simulink model "vvc1phase_simpower"  (Simulink 10.2)
settings: Solver=ode3  StartTime=0.0  StopTime=0.5  FixedStep=.00000005  MaxStep=.0000001  RelTol=1e-3  EnableMultiTasking=on
libraries: powerlib x32, simulink x11
(part 1 of 2)
settings Model: Creator=100004357  LastModifiedBy=bjeppese
settings DataIOCC: LimitDataPoints=on
settings OptimizationCC: ExpressionDepthLimit=2147483647
settings DebuggingCC: SolverPrmCheckMsg=warning  MultiTaskDSMMsg=warning  MultiTaskCondExecSysMsg=none  StateNameClashWarn=warning
settings SimscapeCC: SimscapeNormalizeSystem=off

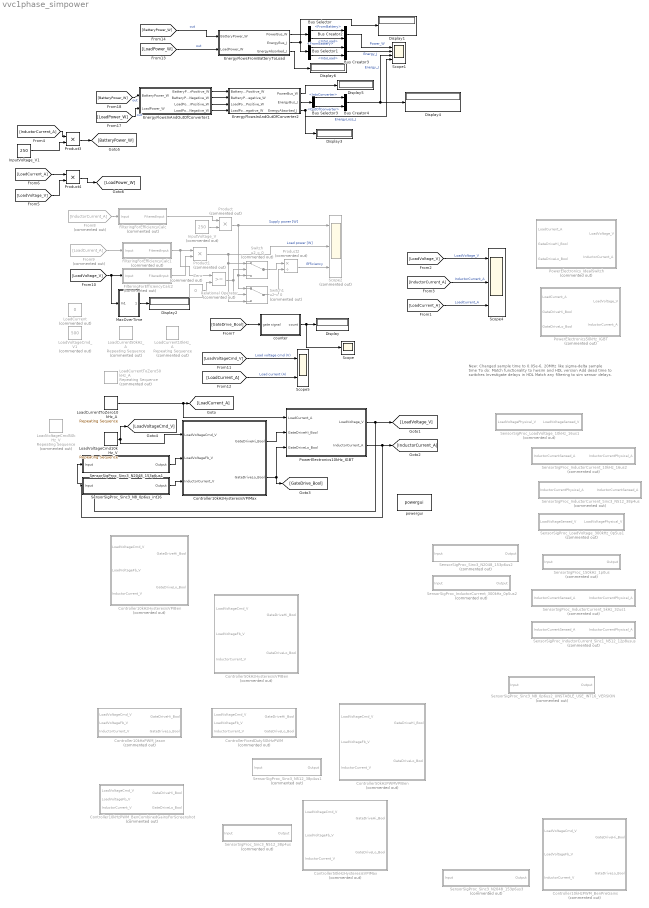
== system vvc1phase_simpower ==
  note: New:
      | Changed sample time to 0.05e-6, 20MHz like sigma-delta sample time
      |
      |
      | To do:
      | Match functionality to hwsim and HDL version
      | Add dead time to switches
      | Investigate delays in HDL
      | Match any filtering to sim sensor delays.
  Bus Creator2 : BusCreator  Inputs=2
  Bus Creator3 : BusCreator  Inputs=2
  Bus Creator4 : BusCreator  Inputs=2
  Bus Selector : BusSelector  OutputSignals=FromBattery,IntoLoad
  Bus Selector1 : BusSelector  OutputSignals=FromBattery,IntoLoad
  Bus Selector3 : BusSelector  OutputSignals=IntoConverter,OutOfConverter
  Controller10kHzHysteresisVPIBen : Subsystem  Commented=on
  Controller10kHzHysteresisVPIMax : Subsystem
  Controller10kHzPWM_BenCombinedGainsForScreenshot : Subsystem  Commented=on
  Controller10kHzPWM_BenPreGains : Subsystem  Commented=on
  "Controller10kHzPWM_Jason " : Subsystem  Commented=on
  Controller50kHzHysteresisVPIBen : Subsystem  Commented=on
  Controller50kHzHysteresisVPIMax : Subsystem  Commented=on
  Controller50kHzPWMVPIBen : Subsystem  Commented=on
  ControllerFixedDuty50kHzPWM : Subsystem  Commented=on
  Display{,1..6} (7 alike) : Display
  EnergyFlowsFromBatteryToLoad : Subsystem
  EnergyFlowsInAndOutOfConverter1 : Subsystem
  EnergyFlowsInAndOutOfConverter2 : Subsystem
  FilteringForEfficiencyCalc : Subsystem  Commented=on
  FilteringForEfficiencyCalc1 : Subsystem  Commented=on
  FilteringForEfficiencyCalc2 : Subsystem  Commented=on
  From8 : From  Commented=on  GotoTag=InductorCurrent_A
  From9 : From  Commented=on  GotoTag=LoadCurrent_A
  InputVoltage_V : Constant  Commented=on  Value=250
  InputVoltage_V1 : Constant  Value=250
  LoadCurrent : Constant  Commented=on  Value=0
  LoadCurrent10kHz_A : simulink/Sources/Repeating Sequence  Commented=on  rep_seq_t=[0 .05 .05001 .100 .10001 .150 .15001 .200 .20001 .250 .25001 .300 .30001 .350 .35001 .400 .40001 .50]  rep_seq_y=[0 0 10 10 -10 -10 20 20 -20 -20 50 50 -50 -50 100 100 -100 -100]
  LoadCurrent50kHz_A : simulink/Sources/Repeating Sequence  Commented=on  rep_seq_t=[0 .01 .01001 .020 .02001 .030 .03001 .040 .04001 .050 .05001 .060 .06001 .070 .07001 .080 .08001 .10]  rep_seq_y=[0 0 10 10 -10 -10 20 20 -20 -20 50 50 -50 -50 100 100 -100 -100]
  LoadCurrentToZero10kHz_A : simulink/Sources/Repeating Sequence  rep_seq_t=[0 .05 .05001 .100 .10001 .150 .15001 .200 .20001 .250 .25001 .300 .30001 .350 .35001 .400 .40001 .450 .45001 .50]  rep_seq_y=[0 0 10 10 -10 -10 20 20 -20 -20 50 50 -50 -50 100 100 -100 -100 0 0]
  LoadCurrentToZero50kHz_A : simulink/Sources/Repeating Sequence  Commented=on  rep_seq_t=[0 .01 .01001 .020 .02001 .030 .03001 .040 .04001 .050 .05001 .060 .06001 .070 .07001 .080 .08001 .090 .09001 .10]  rep_seq_y=[0 0 10 10 -10 -10 20 20 -20 -20 50 50 -50 -50 100 100 -100 -100 0 0]
  LoadVoltageCmd10kHz_V : simulink/Sources/Repeating Sequence  rep_seq_t=[0 0.00501 0.00502 .450 .45001 .50]  rep_seq_y=[250 250 500 500 250 250]
  LoadVoltageCmd50kHz_V : simulink/Sources/Repeating Sequence  Commented=on  rep_seq_t=[0 0.00101 0.00102 .090 .09001 .10]  rep_seq_y=[250 250 500 500 250 250]
  LoadVoltageCmd_V1 : Constant  Commented=on  Value=500
  MaxOverTime : Subsystem
  PowerElectronics10kHz_IGBT : Subsystem
  PowerElectronics50kHz_IGBT : Subsystem  Commented=on
  PowerElectronics_IdealSwitch : Subsystem  Commented=on
  Product : Product  Commented=on
  Product1 : Product  Commented=on
  Product2 : Product  Commented=on  Inputs=*/
  Product3 : Product
  Product4 : Product
  Relational Operator : RelationalOperator  Commented=on  OutDataTypeStr=boolean  RndMeth=Nearest
  Scope : Scope
  Scope1 : Scope  NumInputPorts=4
  Scope2 : Scope  Commented=on  NumInputPorts=3
  Scope4 : Scope  NumInputPorts=3
  Scope5 : Scope  NumInputPorts=2
  SensorSigProc_150kHz_1p0us : Subsystem  Commented=on
  SensorSigProc_InductorCurrent_10kHz_16us2 : Subsystem  Commented=on
  SensorSigProc_InductorCurrent_300kHz_0p5us2 : Subsystem  Commented=on
  SensorSigProc_InductorCurrent_5kHz_32us1 : Subsystem  Commented=on
  SensorSigProc_InductorCurrent_Sinc1_N512_12p8usus : Subsystem  Commented=on
  SensorSigProc_InductorCurrent_Sinc3_N512_38p4us : Subsystem  Commented=on
  SensorSigProc_LoadVoltage_10kHz_16us1 : Subsystem  Commented=on
  SensorSigProc_LoadVoltage_300kHz_0p5us1 : Subsystem  Commented=on
  SensorSigProc_Sinc3_N2048_153p6us1 : Subsystem
  SensorSigProc_Sinc3_N2048_153p6us2 : Subsystem  Commented=on
  SensorSigProc_Sinc3_N2048_153p6us3 : Subsystem  Commented=on
  SensorSigProc_Sinc3_N512_38p4us : Subsystem  Commented=on
  SensorSigProc_Sinc3_N512_38p4us1 : Subsystem  Commented=on
  SensorSigProc_Sinc3_N8_0p6us2_UNSTABLE_USE_INT16_VERSION : Subsystem  Commented=on
  SensorSigProc_Sinc3_N8_0p6us_int16 : Subsystem
  Switch : Switch  Commented=on  Criteria=u2 > Threshold
  Switch1 : Switch  Commented=on  Criteria=u2 > Threshold
  Zero : Constant  Commented=on  Value=0
  "counter " : Subsystem
  powergui : powerlib/powergui  Priority=1  SimulationMode=Discrete  SampleTime=5e-8  frequency=60  Iterations=50  frequencyindice=0  Pbase=100e6  ErrMax=1e-4  UnitsV=kV  UnitsW=MW  buscounter=0  FunctionMessages=off  echomessages=off  EnableUseOfTLC=off  CurrentSourceSwitches=off  DisableSnubberDevices=off  DisableRonSwitches=off  DisableVfSwitches=off  DisplayEquations=off  AutomaticDiscreteSolvers=off  SolverType=Tustin  Interpol=off  ExternalGateDelay=off  methode=off  Ts=0  x0status=blocks  SPID=off  SwTol=0  HookPort=off  NonlinearTolerance=1e-4  nMaxIteration=100  ContinueOnMaxIteration=off  RestoreLinks=warning  ResistiveCurrentMeasurement=off  Frange=[0:2:500]  Ylog=off  Xlog=on  ShowGrid=off  save=off  variable=ZData  structure=0  ZoomFFT=off  StartTime=0.0  cycles=1  DisplayStyle=1  fundamental=60  FreqAxis=off  MaxFrequency=1000  frequencyindicesteady=1  RmsSteady=1  display=off
  wires:
  From8/1 -> FilteringForEfficiencyCalc/1(Input)
  InputVoltage_V/1 -> Product/2
  Product/1 -> Switch1/1, Switch/3, Scope2/1  "Supply power [W]"
  From9/1 -> FilteringForEfficiencyCalc1/1(Input)
  [LoadVoltage_V] -> MaxOverTime/1(In1), FilteringForEfficiencyCalc2/1(Input)
  Product1/1 -> Switch1/3, Switch/1, Scope2/2  "Load power [W]"
  Product2/1 -> Scope2/3  "Efficiency"
  LoadVoltageCmd10kHz_V/1 -> Controller10kHzHysteresisVPIMax/1(LoadVoltageCmd_V), [LoadVoltageCmd_V]
  PowerElectronics10kHz_IGBT/1(LoadVoltage_V) -> SensorSigProc_Sinc3_N2048_153p6us1/1(Input), [LoadVoltage_V]
  PowerElectronics10kHz_IGBT/2(InductorCurrent_A) -> SensorSigProc_Sinc3_N8_0p6us_int16/1(Input), [InductorCurrent_A]
  [LoadCurrent_A] -> Scope4/3  "LoadCurrent_A"
  [LoadVoltage_V] -> Scope4/1  "LoadVoltage_V"
  [InductorCurrent_A] -> Scope4/2  "InductorCurrent_A"
  FilteringForEfficiencyCalc/1(FiteredInput) -> Product/1
  FilteringForEfficiencyCalc1/1(FiteredInput) -> Relational Operator/1, Product1/1
  FilteringForEfficiencyCalc2/1(FiteredInput) -> Product1/2
  Controller10kHzHysteresisVPIMax/2(GateDriveLo_Bool) -> [GateDrive_Bool], PowerElectronics10kHz_IGBT/3(GateDriveLo_Bool)
  Zero/1 -> Relational Operator/2
  Relational Operator/1 -> Switch/2, Switch1/2
  Switch/1 -> Product2/1
  Switch1/1 -> Product2/2
  LoadCurrentToZero10kHz_A/1 -> PowerElectronics10kHz_IGBT/1(LoadCurrent_A), [LoadCurrent_A]
  "counter "/1(count) -> Scope/1, Display/1
  [GateDrive_Bool] -> "counter "/1(gate signal)
  Controller10kHzHysteresisVPIMax/1(GateDriveHi_Bool) -> PowerElectronics10kHz_IGBT/2(GateDriveHi_Bool)
  SensorSigProc_Sinc3_N2048_153p6us1/1(Output) -> Controller10kHzHysteresisVPIMax/2(LoadVoltageFb_V)
  SensorSigProc_Sinc3_N8_0p6us_int16/1(Output) -> Controller10kHzHysteresisVPIMax/3(InductorCurrent_V)
  [LoadVoltageCmd_V] -> Scope5/1  "Load voltage cmd (V)"
  [LoadCurrent_A] -> Scope5/2  "Load current (A)"
  [LoadCurrent_A] -> Product4/1
  [LoadVoltage_V] -> Product4/2
  Product4/1 -> [LoadPower_W]
  InputVoltage_V1/1 -> Product3/2
  [InductorCurrent_A] -> Product3/1
  Product3/1 -> [BatteryPower_W]
  EnergyFlowsFromBatteryToLoad/2(EnergyBus_J) -> Bus Selector1/1, Display1/1
  [BatteryPower_W] -> EnergyFlowsFromBatteryToLoad/1(BatteryPower_W)  "out"
  [LoadPower_W] -> EnergyFlowsFromBatteryToLoad/2(LoadPower_W)  "out"
  [BatteryPower_W] -> EnergyFlowsInAndOutOfConverter1/1(BatteryPower_W)  "out"
  [LoadPower_W] -> EnergyFlowsInAndOutOfConverter1/2(LoadPower_W)  "out"
  EnergyFlowsInAndOutOfConverter1/4(LoadPowerNegative_W) -> EnergyFlowsInAndOutOfConverter2/4(LoadPowerNegative_W)
  EnergyFlowsInAndOutOfConverter1/1(BatteryPowerPositive_W) -> EnergyFlowsInAndOutOfConverter2/1(BatteryPowerPositive_W)
  EnergyFlowsInAndOutOfConverter1/2(BatteryPowerNegative_W) -> EnergyFlowsInAndOutOfConverter2/2(BatteryPowerNegative_W)
  EnergyFlowsInAndOutOfConverter1/3(LoadPowerPositive_W) -> EnergyFlowsInAndOutOfConverter2/3(LoadPowerPositive_W)
  EnergyFlowsFromBatteryToLoad/1(PowerBus_W) -> Bus Selector/1
  Bus Selector/2 -> Bus Creator2/2  "<IntoLoad>"
  Bus Selector/1 -> Bus Creator2/1  "<FromBattery>"
  Bus Creator2/1 -> Scope1/1  "Power_W"
  Bus Selector1/1 -> Bus Creator3/1  "<FromBattery>"
  Bus Selector1/2 -> Bus Creator3/2  "<IntoLoad>"
  Bus Creator3/1 -> Scope1/2  "Energy_J"
  EnergyFlowsInAndOutOfConverter2/2(EnergyBus_J) -> Bus Selector3/1
  Bus Selector3/2 -> Bus Creator4/2  "<OutOfConverter>"
  Bus Creator4/1 -> Scope1/3, Display4/1  "Energy_J"
  Bus Selector3/1 -> Bus Creator4/1  "<IntoConverter>"
  EnergyFlowsInAndOutOfConverter2/3(EnergyAbsorbed_J) -> Scope1/4, Display3/1  "EnergyLoss_J"
  EnergyFlowsInAndOutOfConverter2/1(PowerBus_W) -> Display5/1
  EnergyFlowsFromBatteryToLoad/3(EnergyAbsorbed_J) -> Display6/1
  MaxOverTime/1(Out1) -> Display2/1

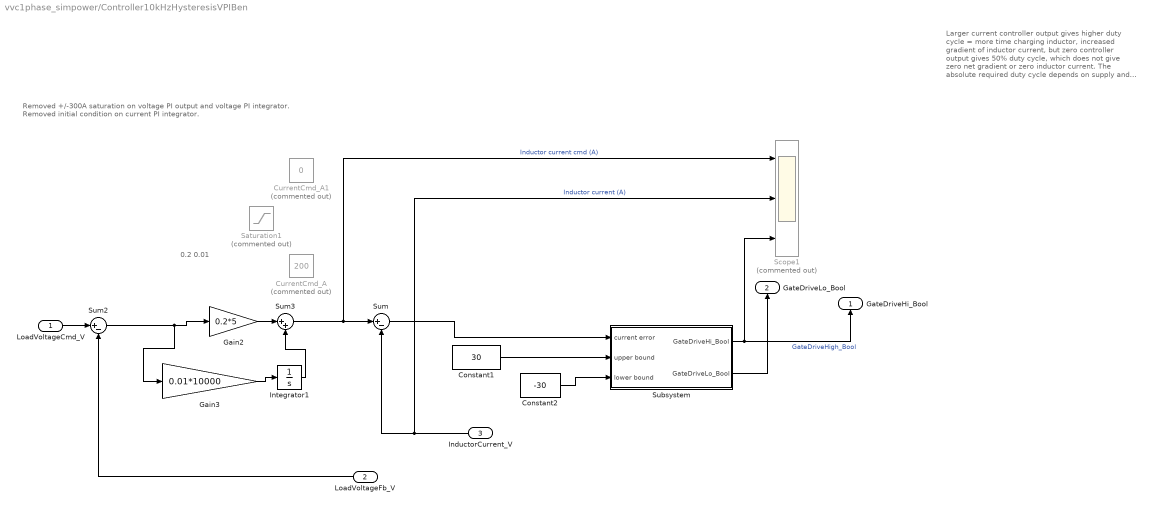
== system vvc1phase_simpower/Controller10kHzHysteresisVPIBen ==
  note: Removed +/-300A saturation on voltage PI output and voltage PI integrator.
      | Removed initial condition on current PI integrator.
  note: Larger current controller output gives higher duty
      | cycle = more time charging inductor,
      | increased gradient of inductor current,
      | but zero controller output gives 50% duty cycle,
      | which does not give zero net gradient
      | or zero inductor current.
      |
      | The absolute required duty cycle depends on
      | supply and load voltages (known)
      | and load current  (unknown)
      | as well as inductor current error.
      |
      | On switch on, with 250V at supply and load,
      | a minimum duty cycle (-0.99) is required to
      | achieve an initial zero inductor current.
      |
      | If zero (50%) were applied initially,
      | inductor current will quickly rise because there
      | is no net voltage reducing it when the inductor
      | is connector to the load. The integrator initial
      | value is used to achieve this.
      |
      | Once the 500V load voltage demand is applied,
      | the voltage controller will give a positive
      | inductor current command.
      | the current P and I gains will raise the duty cycle
      | and the integrator will rise towards zero.
      |
      | Current controller tends to oscillate because
      | controller output only affects gradient of
      | inductor current. Would probably be better
      | with a derivative term
  note: 0.2
      | 0.01
  LoadVoltageCmd_V : Inport
  LoadVoltageFb_V : Inport  Port=2
  InductorCurrent_V : Inport  Port=3
  Constant1 : Constant  Value=30
  Constant2 : Constant  Value=-30
  CurrentCmd_A : Constant  Commented=on  Value=200
  CurrentCmd_A1 : Constant  Commented=on  Value=0
  Gain2 : Gain  Gain=0.2*5
  Gain3 : Gain  Gain=0.01*10000
  Integrator1 : Integrator  UpperSaturationLimit=300  LowerSaturationLimit=-300
  Saturation1 : Saturate  Commented=on  UpperLimit=300  LowerLimit=-300
  Scope1 : Scope  Commented=on  NumInputPorts=3
  Subsystem : Subsystem
  Sum : Sum  Inputs=|+-
  Sum2 : Sum  Inputs=|+-
  Sum3 : Sum  Inputs=|++
  GateDriveHi_Bool : Outport
  GateDriveLo_Bool : Outport  Port=2
  wires:
  Sum3/1 -> Scope1/1, Sum/1  "Inductor current cmd (A)"
  Sum2/1 -> Gain3/1, Gain2/1
  Sum/1 -> Subsystem/1(current error)
  Gain3/1 -> Integrator1/1
  LoadVoltageCmd_V/1 -> Sum2/1
  Integrator1/1 -> Sum3/2
  LoadVoltageFb_V/1 -> Sum2/2
  InductorCurrent_V/1 -> Scope1/2, Sum/2  "Inductor current (A)"
  Gain2/1 -> Sum3/1
  Constant2/1 -> Subsystem/3(lower bound)
  Constant1/1 -> Subsystem/2(upper bound)
  Subsystem/1(GateDriveHi_Bool) -> Scope1/3, GateDriveHi_Bool/1  "GateDriveHigh_Bool"
  Subsystem/2(GateDriveLo_Bool) -> GateDriveLo_Bool/1

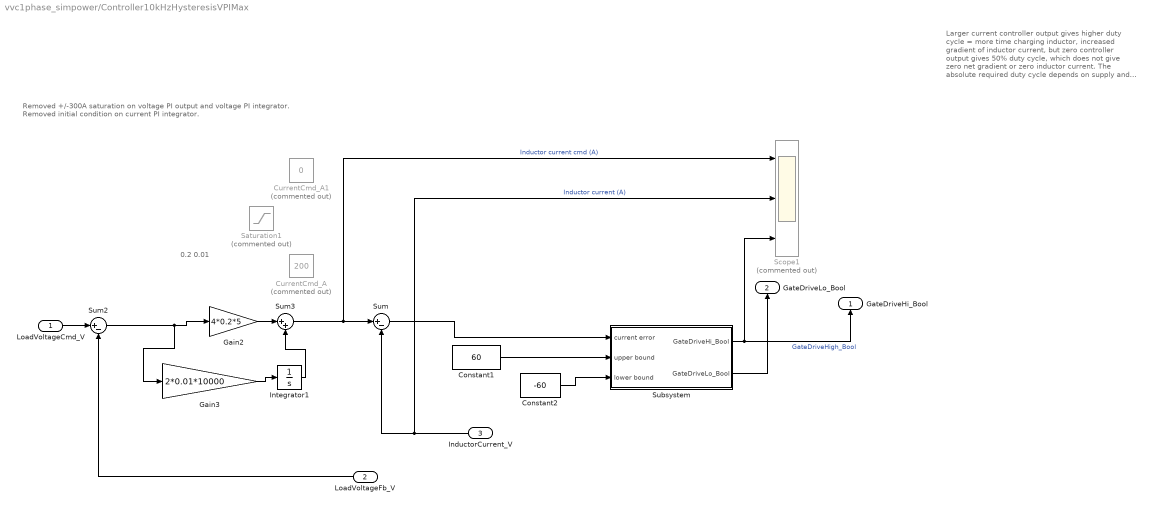
== system vvc1phase_simpower/Controller10kHzHysteresisVPIMax ==
  note: 0.2
      | 0.01
  note: Larger current controller output gives higher duty
      | cycle = more time charging inductor,
      | increased gradient of inductor current,
      | but zero controller output gives 50% duty cycle,
      | which does not give zero net gradient
      | or zero inductor current.
      |
      | The absolute required duty cycle depends on
      | supply and load voltages (known)
      | and load current  (unknown)
      | as well as inductor current error.
      |
      | On switch on, with 250V at supply and load,
      | a minimum duty cycle (-0.99) is required to
      | achieve an initial zero inductor current.
      |
      | If zero (50%) were applied initially,
      | inductor current will quickly rise because there
      | is no net voltage reducing it when the inductor
      | is connector to the load. The integrator initial
      | value is used to achieve this.
      |
      | Once the 500V load voltage demand is applied,
      | the voltage controller will give a positive
      | inductor current command.
      | the current P and I gains will raise the duty cycle
      | and the integrator will rise towards zero.
      |
      | Current controller tends to oscillate because
      | controller output only affects gradient of
      | inductor current. Would probably be better
      | with a derivative term
  note: Removed +/-300A saturation on voltage PI output and voltage PI integrator.
      | Removed initial condition on current PI integrator.
  LoadVoltageCmd_V : Inport
  LoadVoltageFb_V : Inport  Port=2
  InductorCurrent_V : Inport  Port=3
  Constant1 : Constant  Value=60
  Constant2 : Constant  Value=-60
  CurrentCmd_A : Constant  Commented=on  Value=200
  CurrentCmd_A1 : Constant  Commented=on  Value=0
  Gain2 : Gain  Gain=4*0.2*5
  Gain3 : Gain  Gain=2*0.01*10000
  Integrator1 : Integrator  UpperSaturationLimit=300  LowerSaturationLimit=-300
  Saturation1 : Saturate  Commented=on  UpperLimit=300  LowerLimit=-300
  Scope1 : Scope  Commented=on  NumInputPorts=3
  Subsystem : Subsystem
  Sum : Sum  Inputs=|+-
  Sum2 : Sum  Inputs=|+-
  Sum3 : Sum  Inputs=|++
  GateDriveHi_Bool : Outport
  GateDriveLo_Bool : Outport  Port=2
  wires:
  Subsystem/2(GateDriveLo_Bool) -> GateDriveLo_Bool/1
  Subsystem/1(GateDriveHi_Bool) -> GateDriveHi_Bool/1, Scope1/3  "GateDriveHigh_Bool"
  Constant1/1 -> Subsystem/2(upper bound)
  Constant2/1 -> Subsystem/3(lower bound)
  Gain2/1 -> Sum3/1
  InductorCurrent_V/1 -> Sum/2, Scope1/2  "Inductor current (A)"
  LoadVoltageFb_V/1 -> Sum2/2
  Integrator1/1 -> Sum3/2
  LoadVoltageCmd_V/1 -> Sum2/1
  Gain3/1 -> Integrator1/1
  Sum/1 -> Subsystem/1(current error)
  Sum2/1 -> Gain2/1, Gain3/1
  Sum3/1 -> Sum/1, Scope1/1  "Inductor current cmd (A)"

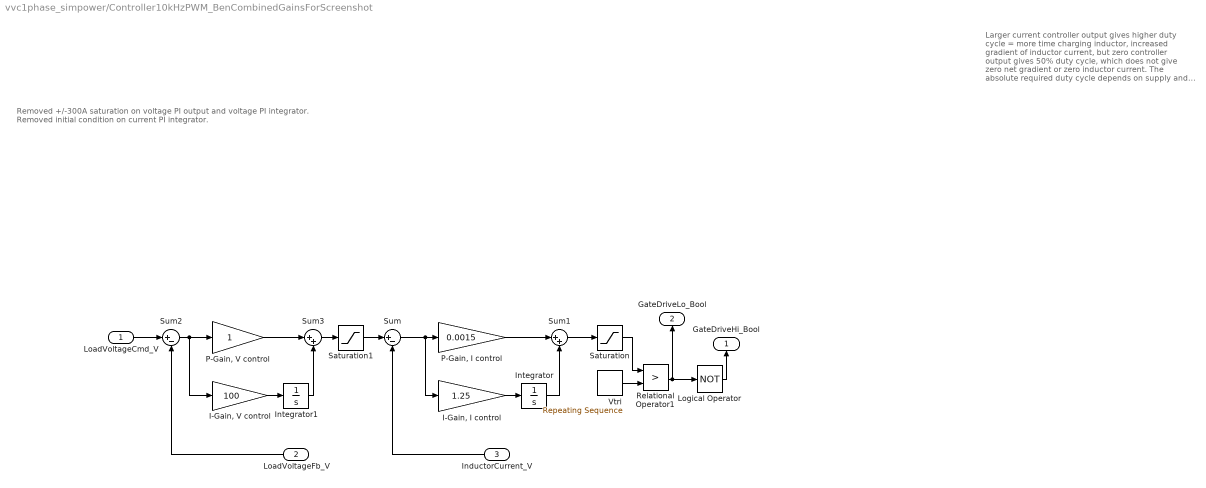
== system vvc1phase_simpower/Controller10kHzPWM_BenCombinedGainsForScreenshot ==
  note: Removed +/-300A saturation on voltage PI output and voltage PI integrator.
      | Removed initial condition on current PI integrator.
  note: Larger current controller output gives higher duty
      | cycle = more time charging inductor,
      | increased gradient of inductor current,
      | but zero controller output gives 50% duty cycle,
      | which does not give zero net gradient
      | or zero inductor current.
      |
      | The absolute required duty cycle depends on
      | supply and load voltages (known)
      | and load current  (unknown)
      | as well as inductor current error.
      |
      | On switch on, with 250V at supply and load,
      | a minimum duty cycle (-0.99) is required to
      | achieve an initial zero inductor current.
      |
      | If zero (50%) were applied initially,
      | inductor current will quickly rise because there
      | is no net voltage reducing it when the inductor
      | is connector to the load. The integrator initial
      | value is used to achieve this.
      |
      | Once the 500V load voltage demand is applied,
      | the voltage controller will give a positive
      | inductor current command.
      | the current P and I gains will raise the duty cycle
      | and the integrator will rise towards zero.
      |
      | Current controller tends to oscillate because
      | controller output only affects gradient of
      | inductor current. Would probably be better
      | with a derivative term
  LoadVoltageCmd_V : Inport
  LoadVoltageFb_V : Inport  Port=2
  InductorCurrent_V : Inport  Port=3
  "I-Gain, I control" : Gain  Gain=1.25
  "I-Gain, V control" : Gain  Gain=100
  Integrator : Integrator  InitialCondition=-0.99  LimitOutput=on  UpperSaturationLimit=.99  LowerSaturationLimit=-.99
  Integrator1 : Integrator  LimitOutput=on  UpperSaturationLimit=300  LowerSaturationLimit=-300
  Logical Operator : Logic  Operator=NOT  AllPortsSameDT=off  OutDataTypeStr=boolean
  "P-Gain, I control" : Gain  Gain=0.0015
  "P-Gain, V control" : Gain
  Relational Operator1 : RelationalOperator  Operator=>  OutDataTypeStr=boolean  RndMeth=Nearest
  Saturation : Saturate  UpperLimit=.99  LowerLimit=-.99
  Saturation1 : Saturate  UpperLimit=300  LowerLimit=-300
  Sum : Sum  Inputs=|+-
  Sum1 : Sum  Inputs=|++
  Sum2 : Sum  Inputs=|+-
  Sum3 : Sum  Inputs=|++
  Vtri : simulink/Sources/Repeating Sequence  rep_seq_t=[0 1/20000 1/10000 ]  rep_seq_y=[-1 1 -1]
  GateDriveHi_Bool : Outport
  GateDriveLo_Bool : Outport  Port=2
  wires:
  Sum3/1 -> Saturation1/1
  Sum2/1 -> "P-Gain, V control"/1, "I-Gain, V control"/1
  Sum/1 -> "I-Gain, I control"/1, "P-Gain, I control"/1
  "I-Gain, V control"/1 -> Integrator1/1
  Logical Operator/1 -> GateDriveHi_Bool/1
  LoadVoltageCmd_V/1 -> Sum2/1
  Integrator1/1 -> Sum3/2
  Integrator/1 -> Sum1/2
  "I-Gain, I control"/1 -> Integrator/1
  Relational Operator1/1 -> Logical Operator/1, GateDriveLo_Bool/1
  "P-Gain, I control"/1 -> Sum1/1
  Saturation/1 -> Relational Operator1/1
  Sum1/1 -> Saturation/1
  LoadVoltageFb_V/1 -> Sum2/2
  InductorCurrent_V/1 -> Sum/2
  Vtri/1 -> Relational Operator1/2
  "P-Gain, V control"/1 -> Sum3/1
  Saturation1/1 -> Sum/1

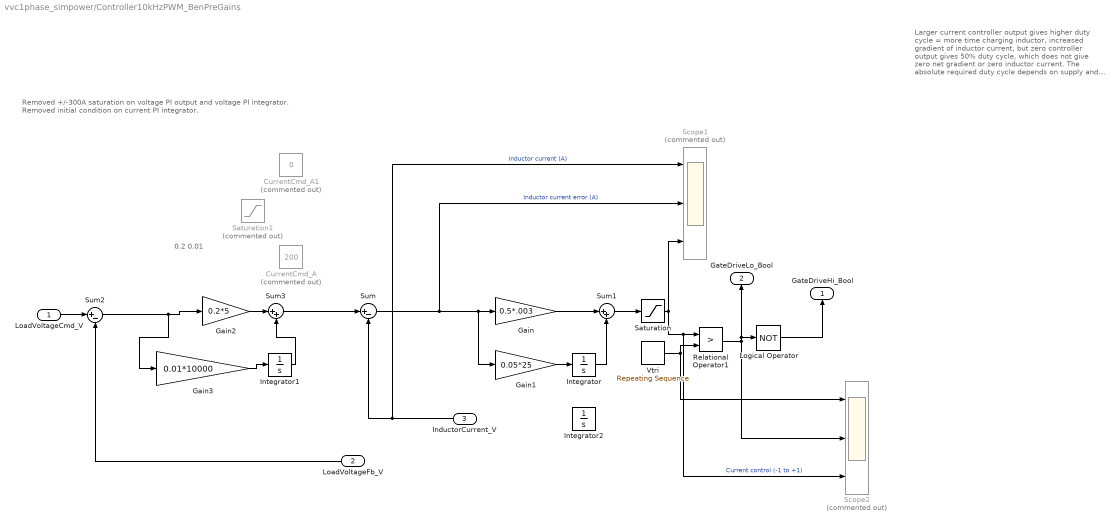
== system vvc1phase_simpower/Controller10kHzPWM_BenPreGains ==
  note: 0.2
      | 0.01
  note: Larger current controller output gives higher duty
      | cycle = more time charging inductor,
      | increased gradient of inductor current,
      | but zero controller output gives 50% duty cycle,
      | which does not give zero net gradient
      | or zero inductor current.
      |
      | The absolute required duty cycle depends on
      | supply and load voltages (known)
      | and load current  (unknown)
      | as well as inductor current error.
      |
      | On switch on, with 250V at supply and load,
      | a minimum duty cycle (-0.99) is required to
      | achieve an initial zero inductor current.
      |
      | If zero (50%) were applied initially,
      | inductor current will quickly rise because there
      | is no net voltage reducing it when the inductor
      | is connector to the load. The integrator initial
      | value is used to achieve this.
      |
      | Once the 500V load voltage demand is applied,
      | the voltage controller will give a positive
      | inductor current command.
      | the current P and I gains will raise the duty cycle
      | and the integrator will rise towards zero.
      |
      | Current controller tends to oscillate because
      | controller output only affects gradient of
      | inductor current. Would probably be better
      | with a derivative term
  note: Removed +/-300A saturation on voltage PI output and voltage PI integrator.
      | Removed initial condition on current PI integrator.
  LoadVoltageCmd_V : Inport
  LoadVoltageFb_V : Inport  Port=2
  InductorCurrent_V : Inport  Port=3
  CurrentCmd_A : Constant  Commented=on  Value=200
  CurrentCmd_A1 : Constant  Commented=on  Value=0
  Gain : Gain  Gain=0.5*.003
  Gain1 : Gain  Gain=0.05*25
  Gain2 : Gain  Gain=0.2*5
  Gain3 : Gain  Gain=0.01*10000
  Integrator : Integrator  InitialCondition=-0.99  LimitOutput=on  UpperSaturationLimit=.99  LowerSaturationLimit=-.99
  Integrator1 : Integrator  UpperSaturationLimit=300  LowerSaturationLimit=-300
  Integrator2 : Integrator  InitialCondition=-.99  LimitOutput=on  UpperSaturationLimit=.99  LowerSaturationLimit=-.99
  Logical Operator : Logic  Operator=NOT  AllPortsSameDT=off  OutDataTypeStr=boolean
  Relational Operator1 : RelationalOperator  Operator=>  OutDataTypeStr=boolean  RndMeth=Nearest
  Saturation : Saturate  UpperLimit=.99  LowerLimit=-.99
  Saturation1 : Saturate  Commented=on  UpperLimit=300  LowerLimit=-300
  Scope1 : Scope  Commented=on  NumInputPorts=3
  Scope2 : Scope  Commented=on  NumInputPorts=3
  Sum : Sum  Inputs=|+-
  Sum1 : Sum  Inputs=|++
  Sum2 : Sum  Inputs=|+-
  Sum3 : Sum  Inputs=|++
  Vtri : simulink/Sources/Repeating Sequence  rep_seq_t=[0 1/20000 1/10000 ]  rep_seq_y=[-1 1 -1]
  GateDriveHi_Bool : Outport
  GateDriveLo_Bool : Outport  Port=2
  wires:
  Gain2/1 -> Sum3/1
  Vtri/1 -> Relational Operator1/2, Scope2/1
  InductorCurrent_V/1 -> Scope1/1, Sum/2  "Inductor current (A)"
  LoadVoltageFb_V/1 -> Sum2/2
  Sum1/1 -> Saturation/1
  Saturation/1 -> Scope1/3, Scope2/3, Relational Operator1/1  "Current control (-1 to +1)"
  Gain/1 -> Sum1/1
  Relational Operator1/1 -> GateDriveLo_Bool/1, Logical Operator/1, Scope2/2
  Gain1/1 -> Integrator/1
  Integrator/1 -> Sum1/2
  Integrator1/1 -> Sum3/2
  LoadVoltageCmd_V/1 -> Sum2/1
  Logical Operator/1 -> GateDriveHi_Bool/1
  Gain3/1 -> Integrator1/1
  Sum/1 -> Scope1/2, Gain1/1, Gain/1  "Inductor current error (A)"
  Sum2/1 -> Gain2/1, Gain3/1
  Sum3/1 -> Sum/1

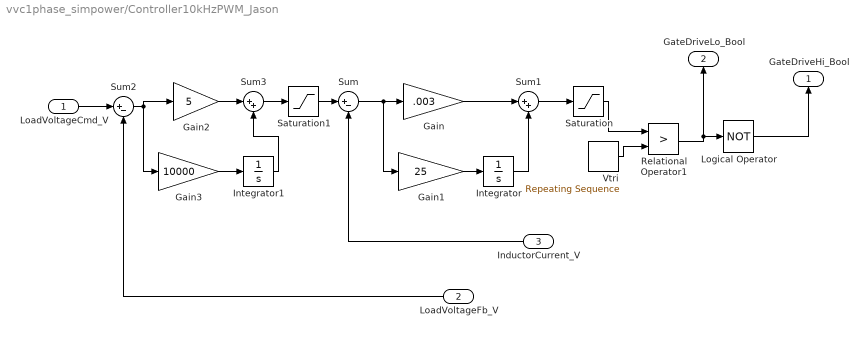
== system vvc1phase_simpower/Controller10kHzPWM_Jason  ==
  LoadVoltageCmd_V : Inport
  LoadVoltageFb_V : Inport  Port=2
  InductorCurrent_V : Inport  Port=3
  Gain : Gain  Gain=.003
  Gain1 : Gain  Gain=25
  Gain2 : Gain  Gain=5
  Gain3 : Gain  Gain=10000
  Integrator : Integrator  InitialCondition=-.99  LimitOutput=on  UpperSaturationLimit=.99  LowerSaturationLimit=-.99
  Integrator1 : Integrator  LimitOutput=on  UpperSaturationLimit=300  LowerSaturationLimit=-300
  Logical Operator : Logic  Operator=NOT  AllPortsSameDT=off  OutDataTypeStr=boolean
  Relational Operator1 : RelationalOperator  Operator=>  OutDataTypeStr=boolean  RndMeth=Nearest
  Saturation : Saturate  UpperLimit=.99  LowerLimit=-.99
  Saturation1 : Saturate  UpperLimit=300  LowerLimit=-300
  Sum : Sum  Inputs=|+-
  Sum1 : Sum  Inputs=|++
  Sum2 : Sum  Inputs=|+-
  Sum3 : Sum  Inputs=|++
  Vtri : simulink/Sources/Repeating Sequence  rep_seq_t=[0 1/20000 1/10000 ]  rep_seq_y=[-1 1 -1]
  GateDriveHi_Bool : Outport
  GateDriveLo_Bool : Outport  Port=2
  wires:
  Gain3/1 -> Integrator1/1
  Logical Operator/1 -> GateDriveHi_Bool/1
  LoadVoltageCmd_V/1 -> Sum2/1
  Integrator1/1 -> Sum3/2
  Integrator/1 -> Sum1/2
  Gain1/1 -> Integrator/1
  Sum2/1 -> Gain2/1, Gain3/1
  Relational Operator1/1 -> GateDriveLo_Bool/1, Logical Operator/1
  Gain/1 -> Sum1/1
  Saturation/1 -> Relational Operator1/1
  Sum1/1 -> Saturation/1
  Saturation1/1 -> Sum/1
  LoadVoltageFb_V/1 -> Sum2/2
  InductorCurrent_V/1 -> Sum/2
  Vtri/1 -> Relational Operator1/2
  Sum/1 -> Gain/1, Gain1/1
  Gain2/1 -> Sum3/1
  Sum3/1 -> Saturation1/1

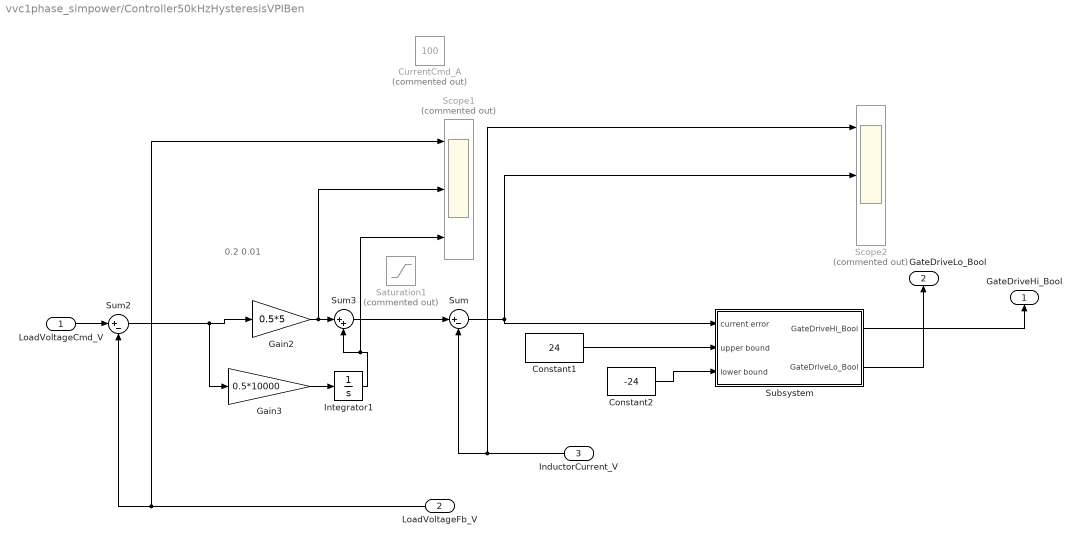
== system vvc1phase_simpower/Controller50kHzHysteresisVPIBen ==
  note: 0.2
      | 0.01
  LoadVoltageCmd_V : Inport
  LoadVoltageFb_V : Inport  Port=2
  InductorCurrent_V : Inport  Port=3
  Constant1 : Constant  Value=24
  Constant2 : Constant  Value=-24
  CurrentCmd_A : Constant  Commented=on  Value=100
  Gain2 : Gain  Gain=0.5*5
  Gain3 : Gain  Gain=0.5*10000
  Integrator1 : Integrator  UpperSaturationLimit=300  LowerSaturationLimit=-300
  Saturation1 : Saturate  Commented=on  UpperLimit=300  LowerLimit=-300
  Scope1 : Scope  Commented=on  NumInputPorts=3
  Scope2 : Scope  Commented=on  NumInputPorts=3
  Subsystem : Subsystem
  Sum : Sum  Inputs=|+-
  Sum2 : Sum  Inputs=|+-
  Sum3 : Sum  Inputs=|++
  GateDriveHi_Bool : Outport
  GateDriveLo_Bool : Outport  Port=2
  wires:
  Subsystem/2(GateDriveLo_Bool) -> GateDriveLo_Bool/1
  Constant1/1 -> Subsystem/2(upper bound)
  Constant2/1 -> Subsystem/3(lower bound)
  Gain2/1 -> Scope1/2, Sum3/1
  InductorCurrent_V/1 -> Scope2/1, Sum/2
  LoadVoltageFb_V/1 -> Scope1/1, Sum2/2
  Integrator1/1 -> Scope1/3, Sum3/2
  LoadVoltageCmd_V/1 -> Sum2/1
  Subsystem/1(GateDriveHi_Bool) -> GateDriveHi_Bool/1
  Gain3/1 -> Integrator1/1
  Sum/1 -> Scope2/2, Subsystem/1(current error)
  Sum2/1 -> Gain2/1, Gain3/1
  Sum3/1 -> Sum/1

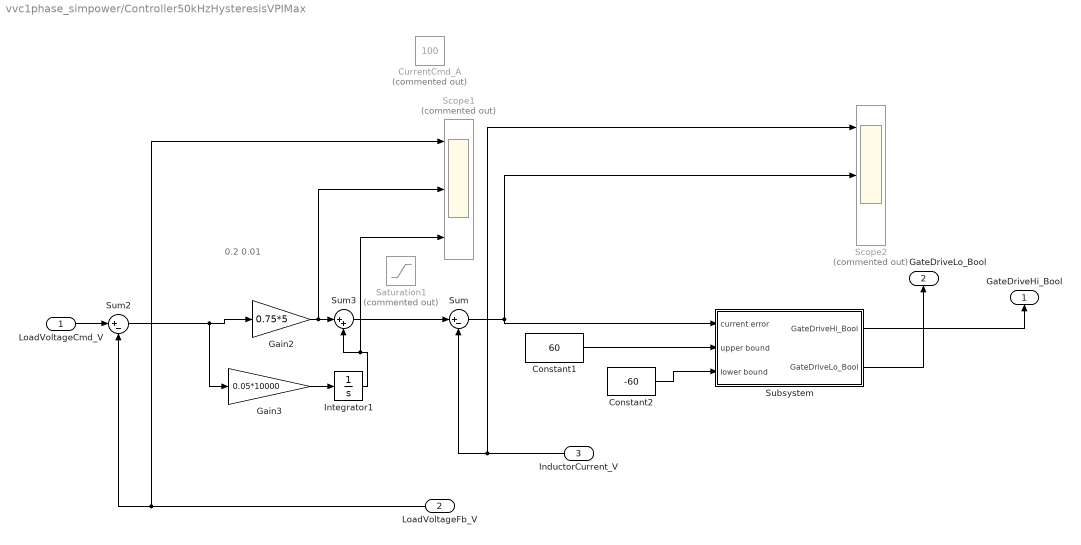
== system vvc1phase_simpower/Controller50kHzHysteresisVPIMax ==
  note: 0.2
      | 0.01
  LoadVoltageCmd_V : Inport
  LoadVoltageFb_V : Inport  Port=2
  InductorCurrent_V : Inport  Port=3
  Constant1 : Constant  Value=60
  Constant2 : Constant  Value=-60
  CurrentCmd_A : Constant  Commented=on  Value=100
  Gain2 : Gain  Gain=0.75*5
  Gain3 : Gain  Gain=0.05*10000
  Integrator1 : Integrator  UpperSaturationLimit=300  LowerSaturationLimit=-300
  Saturation1 : Saturate  Commented=on  UpperLimit=300  LowerLimit=-300
  Scope1 : Scope  Commented=on  NumInputPorts=3
  Scope2 : Scope  Commented=on  NumInputPorts=3
  Subsystem : Subsystem
  Sum : Sum  Inputs=|+-
  Sum2 : Sum  Inputs=|+-
  Sum3 : Sum  Inputs=|++
  GateDriveHi_Bool : Outport
  GateDriveLo_Bool : Outport  Port=2
  wires:
  Sum3/1 -> Sum/1
  Sum2/1 -> Gain3/1, Gain2/1
  Sum/1 -> Subsystem/1(current error), Scope2/2
  Gain3/1 -> Integrator1/1
  Subsystem/1(GateDriveHi_Bool) -> GateDriveHi_Bool/1
  LoadVoltageCmd_V/1 -> Sum2/1
  Integrator1/1 -> Sum3/2, Scope1/3
  LoadVoltageFb_V/1 -> Sum2/2, Scope1/1
  InductorCurrent_V/1 -> Sum/2, Scope2/1
  Gain2/1 -> Sum3/1, Scope1/2
  Constant2/1 -> Subsystem/3(lower bound)
  Constant1/1 -> Subsystem/2(upper bound)
  Subsystem/2(GateDriveLo_Bool) -> GateDriveLo_Bool/1

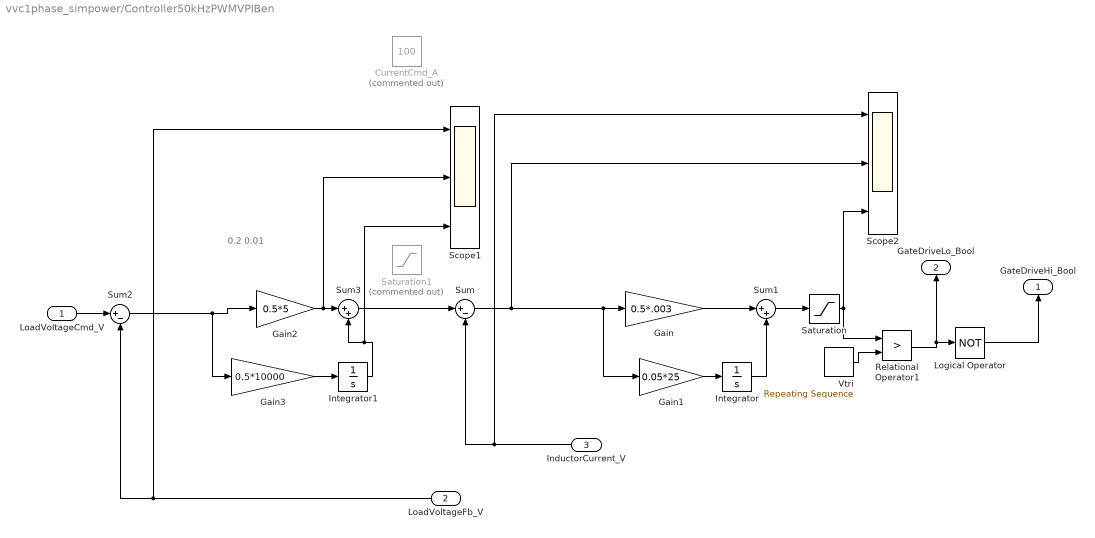
== system vvc1phase_simpower/Controller50kHzPWMVPIBen ==
  note: 0.2
      | 0.01
  LoadVoltageCmd_V : Inport
  LoadVoltageFb_V : Inport  Port=2
  InductorCurrent_V : Inport  Port=3
  CurrentCmd_A : Constant  Commented=on  Value=100
  Gain : Gain  Gain=0.5*.003
  Gain1 : Gain  Gain=0.05*25
  Gain2 : Gain  Gain=0.5*5
  Gain3 : Gain  Gain=0.5*10000
  Integrator : Integrator  InitialCondition=-0.99  LimitOutput=on  UpperSaturationLimit=.99  LowerSaturationLimit=-.99
  Integrator1 : Integrator  UpperSaturationLimit=300  LowerSaturationLimit=-300
  Logical Operator : Logic  Operator=NOT  AllPortsSameDT=off  OutDataTypeStr=boolean
  Relational Operator1 : RelationalOperator  Operator=>  OutDataTypeStr=boolean  RndMeth=Nearest
  Saturation : Saturate  UpperLimit=.99  LowerLimit=-.99
  Saturation1 : Saturate  Commented=on  UpperLimit=300  LowerLimit=-300
  Scope1 : Scope  NumInputPorts=3
  Scope2 : Scope  NumInputPorts=3
  Sum : Sum  Inputs=|+-
  Sum1 : Sum  Inputs=|++
  Sum2 : Sum  Inputs=|+-
  Sum3 : Sum  Inputs=|++
  Vtri : simulink/Sources/Repeating Sequence  rep_seq_t=[0 1/100000 1/50000 ]  rep_seq_y=[-1 1 -1]
  GateDriveHi_Bool : Outport
  GateDriveLo_Bool : Outport  Port=2
  wires:
  Gain2/1 -> Scope1/2, Sum3/1
  Vtri/1 -> Relational Operator1/2
  InductorCurrent_V/1 -> Scope2/1, Sum/2
  LoadVoltageFb_V/1 -> Scope1/1, Sum2/2
  Sum1/1 -> Saturation/1
  Saturation/1 -> Scope2/3, Relational Operator1/1
  Gain/1 -> Sum1/1
  Relational Operator1/1 -> GateDriveLo_Bool/1, Logical Operator/1
  Gain1/1 -> Integrator/1
  Integrator/1 -> Sum1/2
  Integrator1/1 -> Scope1/3, Sum3/2
  LoadVoltageCmd_V/1 -> Sum2/1
  Logical Operator/1 -> GateDriveHi_Bool/1
  Gain3/1 -> Integrator1/1
  Sum/1 -> Scope2/2, Gain1/1, Gain/1
  Sum2/1 -> Gain2/1, Gain3/1
  Sum3/1 -> Sum/1

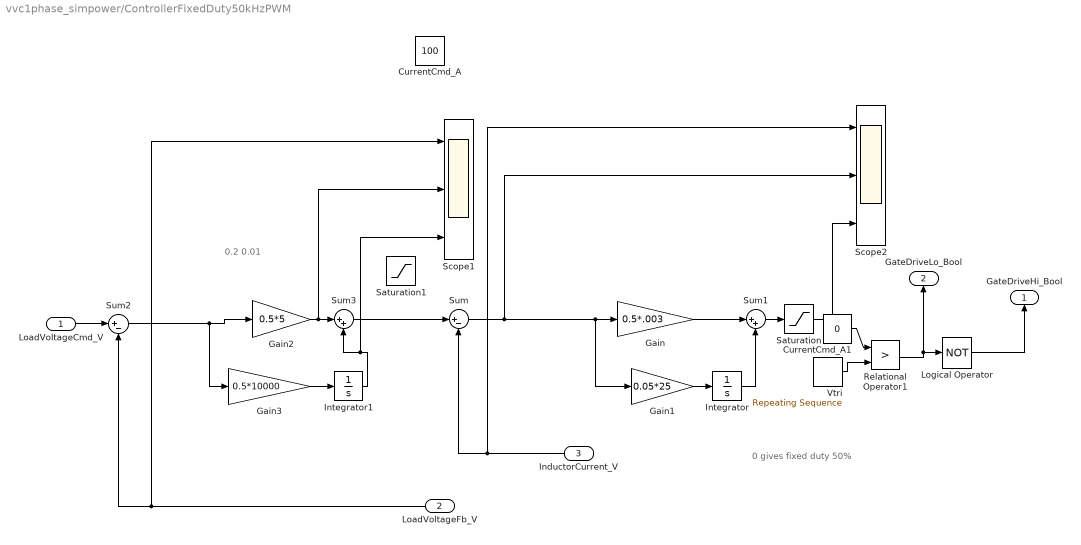
== system vvc1phase_simpower/ControllerFixedDuty50kHzPWM ==
  note: 0 gives fixed duty 50%
  note: 0.2
      | 0.01
  LoadVoltageCmd_V : Inport
  LoadVoltageFb_V : Inport  Port=2
  InductorCurrent_V : Inport  Port=3
  CurrentCmd_A : Constant  Value=100
  CurrentCmd_A1 : Constant  Value=0
  Gain : Gain  Gain=0.5*.003
  Gain1 : Gain  Gain=0.05*25
  Gain2 : Gain  Gain=0.5*5
  Gain3 : Gain  Gain=0.5*10000
  Integrator : Integrator  InitialCondition=-0.99  LimitOutput=on  UpperSaturationLimit=.99  LowerSaturationLimit=-.99
  Integrator1 : Integrator  UpperSaturationLimit=300  LowerSaturationLimit=-300
  Logical Operator : Logic  Operator=NOT  AllPortsSameDT=off  OutDataTypeStr=boolean
  Relational Operator1 : RelationalOperator  Operator=>  OutDataTypeStr=boolean  RndMeth=Nearest
  Saturation : Saturate  UpperLimit=.99  LowerLimit=-.99
  Saturation1 : Saturate  UpperLimit=300  LowerLimit=-300
  Scope1 : Scope  NumInputPorts=3
  Scope2 : Scope  NumInputPorts=3
  Sum : Sum  Inputs=|+-
  Sum1 : Sum  Inputs=|++
  Sum2 : Sum  Inputs=|+-
  Sum3 : Sum  Inputs=|++
  Vtri : simulink/Sources/Repeating Sequence  rep_seq_t=[0 1/100000 1/50000 ]  rep_seq_y=[-1 1 -1]
  GateDriveHi_Bool : Outport
  GateDriveLo_Bool : Outport  Port=2
  wires:
  Sum3/1 -> Sum/1
  Sum2/1 -> Gain3/1, Gain2/1
  Sum/1 -> Gain/1, Gain1/1, Scope2/2
  Gain3/1 -> Integrator1/1
  Logical Operator/1 -> GateDriveHi_Bool/1
  LoadVoltageCmd_V/1 -> Sum2/1
  Integrator1/1 -> Sum3/2, Scope1/3
  Integrator/1 -> Sum1/2
  Gain1/1 -> Integrator/1
  Relational Operator1/1 -> Logical Operator/1, GateDriveLo_Bool/1
  Gain/1 -> Sum1/1
  Saturation/1 -> Scope2/3
  Sum1/1 -> Saturation/1
  LoadVoltageFb_V/1 -> Sum2/2, Scope1/1
  InductorCurrent_V/1 -> Sum/2, Scope2/1
  Vtri/1 -> Relational Operator1/2
  Gain2/1 -> Sum3/1, Scope1/2
  CurrentCmd_A1/1 -> Relational Operator1/1

== system vvc1phase_simpower/EnergyFlowsFromBatteryToLoad ==
  BatteryPower_W : Inport
  LoadPower_W : Inport  Port=2
  Bus Creator : BusCreator  Inputs=2
  Bus Creator1 : BusCreator  Inputs=2
  Integrator : Integrator
  Integrator1 : Integrator
  Sum : Sum  Inputs=|+-
  PowerBus_W : Outport
  EnergyBus_J : Outport  Port=2
  EnergyAbsorbed_J : Outport  Port=3
  wires:
  Integrator1/1 -> Bus Creator1/2, Sum/2  "IntoLoad"
  Bus Creator/1 -> PowerBus_W/1  "Power (W)"
  Bus Creator1/1 -> EnergyBus_J/1  "Energy (J)"
  Sum/1 -> EnergyAbsorbed_J/1  "Energy absorbed (J)"
  Integrator/1 -> Bus Creator1/1, Sum/1  "FromBattery"
  LoadPower_W/1 -> Bus Creator/2, Integrator1/1  "IntoLoad"
  BatteryPower_W/1 -> Integrator/1, Bus Creator/1  "FromBattery"

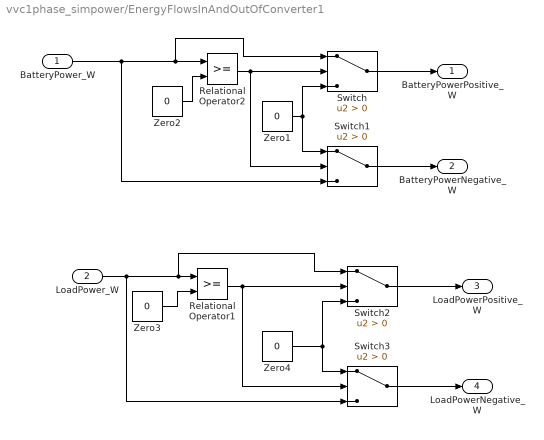
== system vvc1phase_simpower/EnergyFlowsInAndOutOfConverter1 ==
  BatteryPower_W : Inport
  LoadPower_W : Inport  Port=2
  Relational Operator1 : RelationalOperator  OutDataTypeStr=boolean  RndMeth=Nearest
  Relational Operator2 : RelationalOperator  OutDataTypeStr=boolean  RndMeth=Nearest
  Switch{,1..3} (4 alike) : Switch  Criteria=u2 > Threshold
  Zero{1..4} (4 alike) : Constant  Value=0
  BatteryPowerPositive_W : Outport
  BatteryPowerNegative_W : Outport  Port=2
  LoadPowerPositive_W : Outport  Port=3
  LoadPowerNegative_W : Outport  Port=4
  wires:
  Zero4/1 -> Switch2/3, Switch3/1
  Relational Operator1/1 -> Switch2/2, Switch3/2
  Zero3/1 -> Relational Operator1/2
  Zero1/1 -> Switch1/1, Switch/3
  Switch/1 -> BatteryPowerPositive_W/1
  Relational Operator2/1 -> Switch/2, Switch1/2
  Zero2/1 -> Relational Operator2/2
  LoadPower_W/1 -> Switch3/3, Relational Operator1/1, Switch2/1
  BatteryPower_W/1 -> Relational Operator2/1, Switch/1, Switch1/3
  Switch1/1 -> BatteryPowerNegative_W/1
  Switch2/1 -> LoadPowerPositive_W/1
  Switch3/1 -> LoadPowerNegative_W/1

== system vvc1phase_simpower/EnergyFlowsInAndOutOfConverter2 ==
  BatteryPowerPositive_W : Inport
  BatteryPowerNegative_W : Inport  Port=2
  LoadPowerPositive_W : Inport  Port=3
  LoadPowerNegative_W : Inport  Port=4
  Bus Creator : BusCreator  Inputs=2
  Bus Creator1 : BusCreator  Inputs=2
  Integrator : Integrator
  Integrator1 : Integrator
  Sum : Sum  Inputs=|+-
  Sum1 : Sum  Inputs=|+-
  Sum2 : Sum  Inputs=|+-
  PowerBus_W : Outport
  EnergyBus_J : Outport  Port=2
  EnergyAbsorbed_J : Outport  Port=3
  wires:
  Sum2/1 -> Bus Creator/2, Integrator1/1  "OutOfConverter"
  Sum1/1 -> Integrator/1, Bus Creator/1  "IntoConverter"
  Integrator1/1 -> Bus Creator1/2, Sum/2  "OutOfConverter"
  Bus Creator/1 -> PowerBus_W/1  "Power (W)"
  Bus Creator1/1 -> EnergyBus_J/1  "Energy (J)"
  Sum/1 -> EnergyAbsorbed_J/1  "Energy absorbed (J)"
  Integrator/1 -> Bus Creator1/1, Sum/1  "IntoConverter"
  LoadPowerNegative_W/1 -> Sum1/2
  BatteryPowerPositive_W/1 -> Sum1/1
  BatteryPowerNegative_W/1 -> Sum2/2
  LoadPowerPositive_W/1 -> Sum2/1

== system vvc1phase_simpower/FilteringForEfficiencyCalc ==
  note: First order low-pass filter with 200Hz cut-off, time const = 1/(2*pi*f) = 1/(2*pi*200) = 0.0008 = 0.8ms
  Input : Inport
  FilterLowPassFirstOrder200HzCutOff : TransferFcn  Denominator=[0.0008 1]
  FiteredInput : Outport
  wires:
  FilterLowPassFirstOrder200HzCutOff/1 -> FiteredInput/1
  Input/1 -> FilterLowPassFirstOrder200HzCutOff/1

== system vvc1phase_simpower/FilteringForEfficiencyCalc1 ==
  note: First order low-pass filter with 200Hz cut-off, time const = 1/(2*pi*f) = 1/(2*pi*200) = 0.0008 = 0.8ms
  Input : Inport
  FilterLowPassFirstOrder200HzCutOff : TransferFcn  Denominator=[0.0008 1]
  FiteredInput : Outport
  wires:
  Input/1 -> FilterLowPassFirstOrder200HzCutOff/1
  FilterLowPassFirstOrder200HzCutOff/1 -> FiteredInput/1

== system vvc1phase_simpower/FilteringForEfficiencyCalc2 ==
  note: First order low-pass filter with 200Hz cut-off, time const = 1/(2*pi*f) = 1/(2*pi*200) = 0.0008 = 0.8ms
  Input : Inport
  FilterLowPassFirstOrder200HzCutOff : TransferFcn  Denominator=[0.0008 1]
  FiteredInput : Outport
  wires:
  FilterLowPassFirstOrder200HzCutOff/1 -> FiteredInput/1
  Input/1 -> FilterLowPassFirstOrder200HzCutOff/1

== system vvc1phase_simpower/MaxOverTime ==
  In1 : Inport
  Delay1 : Delay  DelayLength=1  InitialCondition=0
  MinMax : MinMax  Function=max  Inputs=2
  Out1 : Outport
  wires:
  MinMax/1 -> Out1/1, Delay1/1
  In1/1 -> MinMax/1
  Delay1/1 -> MinMax/2

== system vvc1phase_simpower/PowerElectronics10kHz_IGBT ==
  LoadCurrent_A : Inport
  GateDriveHi_Bool : Inport  Port=2
  GateDriveLo_Bool : Inport  Port=3
  250 : powerlib/Electrical Sources/DC Voltage Source  Amplitude=250  Measurements=None
  Chv : powerlib/Elements/Series RLC Branch  LConnTagsString=__new0  RConnTagsString=__new0  BranchType=C  Resistance=1  Inductance=1e-3  SetiL0=off  InitialCurrent=0  Capacitance=2000e-6  Setx0=on  InitialVoltage=250  Measurements=None
  Controlled  Current  Source : powerlib/Electrical Sources/Controlled Current Source  Initialize=on  Source_Type=AC  Amplitude=0  Phase=0  Frequency=0  Measurements=None
  Current Measurement1 : powerlib/Measurements/Current Measurement  PhasorSimulation=off  OutputType=Complex  PSBequivalent=0
  Diode1 : powerlib/Power Electronics/Diode  Ron=0.001  Lon=0  Vf=0.8  IC=0  UseSnubber=off  Rs=500  Cs=250e-9  Measurements=off
  Diode2 : powerlib/Power Electronics/Diode  Ron=0.001  Lon=0  Vf=0.8  IC=0  UseSnubber=off  Rs=500  Cs=250e-9  Measurements=off
  Ground : powerlib/Elements/Ground  LConnTagsString=a
  IGBT1 : powerlib/Power Electronics/IGBT  Ron=0.001  Lon=0  Vf=1  Tf=1e-6  Tt=2e-6  IC=0  Rs=1e5  Cs=inf  Measurements=off
  IGBT2 : powerlib/Power Electronics/IGBT  Ron=0.001  Lon=0  Vf=1  Tf=1e-6  Tt=2e-6  IC=0  Rs=1e5  Cs=inf  Measurements=off
  L : powerlib/Elements/Series RLC Branch  LConnTagsString=__new0  RConnTagsString=__new0  BranchType=L  Resistance=35  Inductance=200e-6  SetiL0=on  InitialCurrent=0  Capacitance=1e-6  Setx0=off  InitialVoltage=0  Measurements=None
  Voltage Measurement : powerlib/Measurements/Voltage Measurement  PhasorSimulation=off  OutputType=Complex  PSBequivalent=0
  LoadVoltage_V : Outport
  InductorCurrent_A : Outport  Port=2
  wires:
  GateDriveLo_Bool/1 -> IGBT2/1
  GateDriveHi_Bool/1 -> IGBT1/1
  LoadCurrent_A/1 -> Controlled  Current  Source/1
  Voltage Measurement/1 -> LoadVoltage_V/1  "Output voltage [V]"
  Current Measurement1/1 -> InductorCurrent_A/1  "Inductor current [A]"
  connections:
  Controlled  Current  Source/RConn1 -- Voltage Measurement/LConn2 -- Chv/RConn1 -- Diode2/LConn1 -- IGBT2/RConn1 -- 250/LConn1 -- Ground/LConn1
  Voltage Measurement/LConn1 -- IGBT1/LConn1 -- Diode1/RConn1 -- Chv/LConn1 -- Controlled  Current  Source/LConn1
  250/RConn1 -- L/RConn1
  Current Measurement1/RConn1 -- Diode2/RConn1 -- IGBT2/LConn1 -- Diode1/LConn1 -- IGBT1/RConn1
  L/LConn1 -- Current Measurement1/LConn1

== system vvc1phase_simpower/PowerElectronics50kHz_IGBT ==
  LoadCurrent_A : Inport
  GateDriveHi_Bool : Inport  Port=2
  GateDriveLo_Bool : Inport  Port=3
  250 : powerlib/Electrical Sources/DC Voltage Source  Amplitude=250  Measurements=None
  Chv : powerlib/Elements/Series RLC Branch  LConnTagsString=__new0  RConnTagsString=__new0  BranchType=C  Resistance=1  Inductance=1e-3  SetiL0=off  InitialCurrent=0  Capacitance=400e-6  Setx0=on  InitialVoltage=250  Measurements=None
  Controlled Current Source : powerlib/Electrical Sources/Controlled Current Source  Initialize=on  Source_Type=AC  Amplitude=0  Phase=0  Frequency=0  Measurements=None
  Current Measurement1 : powerlib/Measurements/Current Measurement  PhasorSimulation=off  OutputType=Complex  PSBequivalent=0
  Diode1 : powerlib/Power Electronics/Diode  Ron=0.001  Lon=0  Vf=0.8  IC=0  UseSnubber=off  Rs=500  Cs=250e-9  Measurements=off
  Diode2 : powerlib/Power Electronics/Diode  Ron=0.001  Lon=0  Vf=0.8  IC=0  UseSnubber=off  Rs=500  Cs=250e-9  Measurements=off
  Ground : powerlib/Elements/Ground  LConnTagsString=a
  IGBT1 : powerlib/Power Electronics/IGBT  Ron=0.001  Lon=0  Vf=1  Tf=1e-6  Tt=2e-6  IC=0  Rs=1e5  Cs=inf  Measurements=off
  IGBT2 : powerlib/Power Electronics/IGBT  Ron=0.001  Lon=0  Vf=1  Tf=1e-6  Tt=2e-6  IC=0  Rs=1e5  Cs=inf  Measurements=off
  L : powerlib/Elements/Series RLC Branch  LConnTagsString=__new0  RConnTagsString=__new0  BranchType=L  Resistance=35  Inductance=40e-6  SetiL0=on  InitialCurrent=0  Capacitance=1e-6  Setx0=off  InitialVoltage=0  Measurements=None
  vAN1 : powerlib/Measurements/Voltage Measurement  PhasorSimulation=off  OutputType=Complex  PSBequivalent=0
  LoadVoltage_V : Outport
  InductorCurrent_A : Outport  Port=2
  wires:
  Current Measurement1/1 -> InductorCurrent_A/1  "Inductor current [A]"
  vAN1/1 -> LoadVoltage_V/1  "Output voltage [V]"
  LoadCurrent_A/1 -> Controlled Current Source/1
  GateDriveHi_Bool/1 -> IGBT1/1
  GateDriveLo_Bool/1 -> IGBT2/1
  connections:
  L/LConn1 -- Current Measurement1/LConn1
  IGBT1/RConn1 -- Diode1/LConn1 -- IGBT2/LConn1 -- Diode2/RConn1 -- Current Measurement1/RConn1
  250/RConn1 -- L/RConn1
  Chv/LConn1 -- Controlled Current Source/LConn1 -- IGBT1/LConn1 -- Diode1/RConn1 -- vAN1/LConn1
  Chv/RConn1 -- vAN1/LConn2 -- Ground/LConn1 -- 250/LConn1 -- IGBT2/RConn1 -- Diode2/LConn1 -- Controlled Current Source/RConn1

== system vvc1phase_simpower/PowerElectronics_IdealSwitch ==
  LoadCurrent_A : Inport
  GateDriveHi_Bool : Inport  Port=2
  GateDriveLo_Bool : Inport  Port=3
  250 : powerlib/Electrical Sources/DC Voltage Source  Amplitude=250  Measurements=None
  Chv : powerlib/Elements/Series RLC Branch  LConnTagsString=__new0  RConnTagsString=__new0  BranchType=C  Resistance=1  Inductance=1e-3  SetiL0=off  InitialCurrent=0  Capacitance=400e-6  Setx0=on  InitialVoltage=250  Measurements=None
  Controlled Current Source : powerlib/Electrical Sources/Controlled Current Source  Initialize=on  Source_Type=AC  Amplitude=0  Phase=0  Frequency=0  Measurements=None
  Current Measurement1 : powerlib/Measurements/Current Measurement  PhasorSimulation=off  OutputType=Complex  PSBequivalent=0
  Ground : powerlib/Elements/Ground  LConnTagsString=a
  Ideal Switch1 : powerlib/Power Electronics/Ideal Switch  Ron=0.1  Lon=0  IC=0  Rs=1e3  Cs=inf  Measurements=off
  Ideal Switch2 : powerlib/Power Electronics/Ideal Switch  Ron=0.1  Lon=0  IC=0  Rs=1e3  Cs=inf  Measurements=off
  L : powerlib/Elements/Series RLC Branch  LConnTagsString=__new0  RConnTagsString=__new0  BranchType=L  Resistance=35  Inductance=40e-6  SetiL0=on  InitialCurrent=0  Capacitance=1e-6  Setx0=off  InitialVoltage=0  Measurements=None
  vAN1 : powerlib/Measurements/Voltage Measurement  PhasorSimulation=off  OutputType=Complex  PSBequivalent=0
  LoadVoltage_V : Outport
  InductorCurrent_A : Outport  Port=2
  wires:
  Current Measurement1/1 -> InductorCurrent_A/1  "Inductor current [A]"
  vAN1/1 -> LoadVoltage_V/1  "Output voltage [V]"
  LoadCurrent_A/1 -> Controlled Current Source/1
  GateDriveHi_Bool/1 -> Ideal Switch2/1
  GateDriveLo_Bool/1 -> Ideal Switch1/1
  connections:
  L/LConn1 -- Current Measurement1/LConn1
  Ideal Switch2/LConn1 -- Ideal Switch1/RConn1 -- Current Measurement1/RConn1
  250/RConn1 -- L/RConn1
  Chv/LConn1 -- Controlled Current Source/LConn1 -- Ideal Switch2/RConn1 -- vAN1/LConn1
  Ideal Switch1/LConn1 -- Ground/LConn1 -- 250/LConn1 -- Chv/RConn1 -- vAN1/LConn2 -- Controlled Current Source/RConn1

== system vvc1phase_simpower/SensorSigProc_150kHz_1p0us ==
  note: First order low-pass filter with 150kHz cut-off, time const = 1/(2*pi*f) = 1/(2*pi*150e3) = 1us
  Input : Inport
  FilterLowPassFirstOrder150kHzCutOff : TransferFcn  Denominator=[0.000001 1]
  Output : Outport
  wires:
  FilterLowPassFirstOrder150kHzCutOff/1 -> Output/1
  Input/1 -> FilterLowPassFirstOrder150kHzCutOff/1

== system vvc1phase_simpower/SensorSigProc_InductorCurrent_10kHz_16us2 ==
  note: First order low-pass filter with 10kHz cut-off, time const = 1/(2*pi*f) = 1/(2*pi*10e3) = 1.6e-5 = 16us
  InductorCurrentPhysical_A : Inport
  FilterLowPassFirstOrder10kHzCutOff : TransferFcn  Denominator=[16e-6 1]
  InductorCurrentSensed_A : Outport
  wires:
  InductorCurrentPhysical_A/1 -> FilterLowPassFirstOrder10kHzCutOff/1
  FilterLowPassFirstOrder10kHzCutOff/1 -> InductorCurrentSensed_A/1

== system vvc1phase_simpower/SensorSigProc_InductorCurrent_300kHz_0p5us2 ==
  note: First order low-pass filter with 300kHz cut-off, time const = 1/(2*pi*f) = 1/(2*pi*300e3) = 5e-7 = 0.5us
  Input : Inport
  FilterLowPassFirstOrder300kHzCutOff : TransferFcn  Denominator=[0.0000005 1]
  Output : Outport
  wires:
  Input/1 -> FilterLowPassFirstOrder300kHzCutOff/1
  FilterLowPassFirstOrder300kHzCutOff/1 -> Output/1

== system vvc1phase_simpower/SensorSigProc_InductorCurrent_5kHz_32us1 ==
  note: First order low-pass filter with 5kHz cut-off, time const = 1/(2*pi*f) = 1/(2*pi*5e3) = 3.2e-5 = 32us
  InductorCurrentPhysical_A : Inport
  FilterLowPassFirstOrder5kHzCutOff : TransferFcn  Denominator=[32e-6 1]
  InductorCurrentSensed_A : Outport
  wires:
  FilterLowPassFirstOrder5kHzCutOff/1 -> InductorCurrentSensed_A/1
  InductorCurrentPhysical_A/1 -> FilterLowPassFirstOrder5kHzCutOff/1

== system vvc1phase_simpower/SensorSigProc_InductorCurrent_Sinc1_N512_12p8usus ==
  note: Sinc3, N=512, 20MHz to 39kHz, settling time = 512*0.05e-6=25.6us, delay=12.8us
  InductorCurrentPhysical_A : Inport
  Discrete Integrator : DiscreteFilter  Denominator=[1 -1]
  Discrete differentiator : DiscreteFilter  Numerator=[1 -1]  Denominator=[1]
  Gain : Gain  Gain=1/512
  Rate Transition : RateTransition
  Zero-Order Hold : ZeroOrderHold  SampleTime=512*0.05e-6
  Zero-Order Hold2 : ZeroOrderHold  SampleTime=.00000005
  InductorCurrentSensed_A : Outport
  wires:
  InductorCurrentPhysical_A/1 -> Discrete Integrator/1
  Discrete Integrator/1 -> Zero-Order Hold/1
  Zero-Order Hold/1 -> Discrete differentiator/1
  Discrete differentiator/1 -> Gain/1
  Zero-Order Hold2/1 -> InductorCurrentSensed_A/1
  Rate Transition/1 -> Zero-Order Hold2/1
  Gain/1 -> Rate Transition/1

== system vvc1phase_simpower/SensorSigProc_InductorCurrent_Sinc3_N512_38p4us ==
  note: Sinc3, N=512, 20MHz to 39kHz, settling time = 3*512*0.05e-6=76us, delay=38.4us
  InductorCurrentPhysical_A : Inport
  Discrete Integrator : DiscreteFilter  Denominator=[1 -1]
  Discrete Integrator1 : DiscreteFilter  Denominator=[1 -1]
  Discrete Integrator2 : DiscreteFilter  Denominator=[1 -1]
  Discrete differentiator : DiscreteFilter  Numerator=[1 -1]  Denominator=[1]
  Discrete differentiator1 : DiscreteFilter  Numerator=[1 -1]  Denominator=[1]
  Discrete differentiator2 : DiscreteFilter  Numerator=[1 -1]  Denominator=[1]
  Gain : Gain  Gain=1/512
  Gain1 : Gain  Gain=1/512
  Gain2 : Gain  Gain=1/512
  Rate Transition : RateTransition
  Zero-Order Hold : ZeroOrderHold  SampleTime=512*0.05e-6
  Zero-Order Hold2 : ZeroOrderHold  SampleTime=.00000005
  InductorCurrentSensed_A : Outport
  wires:
  Rate Transition/1 -> Zero-Order Hold2/1
  Zero-Order Hold2/1 -> InductorCurrentSensed_A/1
  Discrete differentiator2/1 -> Gain2/1
  Discrete differentiator1/1 -> Gain1/1
  Discrete differentiator/1 -> Gain/1
  Zero-Order Hold/1 -> Discrete differentiator/1
  Discrete Integrator2/1 -> Zero-Order Hold/1
  Discrete Integrator1/1 -> Discrete Integrator2/1
  Discrete Integrator/1 -> Discrete Integrator1/1
  InductorCurrentPhysical_A/1 -> Discrete Integrator/1
  Gain/1 -> Discrete differentiator1/1
  Gain1/1 -> Discrete differentiator2/1
  Gain2/1 -> Rate Transition/1

== system vvc1phase_simpower/SensorSigProc_LoadVoltage_10kHz_16us1 ==
  LoadVoltagePhysical_V : Inport
  10kHz1 : TransferFcn  Denominator=[16e-6 1]
  LoadVoltageSensed_V : Outport
  wires:
  10kHz1/1 -> LoadVoltageSensed_V/1
  LoadVoltagePhysical_V/1 -> 10kHz1/1

== system vvc1phase_simpower/SensorSigProc_LoadVoltage_300kHz_0p5us1 ==
  LoadVoltagePhysical_V : Inport
  300kHz1 : TransferFcn  Denominator=[0.0000005 1]
  LoadVoltageSensed_V : Outport
  wires:
  300kHz1/1 -> LoadVoltageSensed_V/1
  LoadVoltagePhysical_V/1 -> 300kHz1/1

== system vvc1phase_simpower/SensorSigProc_Sinc3_N2048_153p6us1 ==
  note: Sinc3, N=2048, 20MHz to 9.7kHz, settling time = 3*2048*0.05e-6=307.2us, delay=153.6us
  Input : Inport
  Discrete Integrator : DiscreteFilter  Denominator=[1 -1]
  Discrete Integrator1 : DiscreteFilter  Denominator=[1 -1]
  Discrete Integrator2 : DiscreteFilter  Denominator=[1 -1]
  Discrete differentiator : DiscreteFilter  Numerator=[1 -1]  Denominator=[1]
  Discrete differentiator1 : DiscreteFilter  Numerator=[1 -1]  Denominator=[1]
  Discrete differentiator2 : DiscreteFilter  Numerator=[1 -1]  Denominator=[1]
  Gain : Gain  Gain=1/2048
  Gain1 : Gain  Gain=1/2048
  Gain2 : Gain  Gain=1/2048
  Rate Transition : RateTransition
  Zero-Order Hold : ZeroOrderHold  SampleTime=2048*0.05e-6
  Zero-Order Hold2 : ZeroOrderHold  SampleTime=.00000005
  Output : Outport
  wires:
  Rate Transition/1 -> Zero-Order Hold2/1
  Zero-Order Hold2/1 -> Output/1
  Discrete differentiator2/1 -> Gain2/1
  Discrete differentiator1/1 -> Gain1/1
  Discrete differentiator/1 -> Gain/1
  Zero-Order Hold/1 -> Discrete differentiator/1
  Discrete Integrator2/1 -> Zero-Order Hold/1
  Discrete Integrator1/1 -> Discrete Integrator2/1
  Discrete Integrator/1 -> Discrete Integrator1/1
  Input/1 -> Discrete Integrator/1
  Gain/1 -> Discrete differentiator1/1
  Gain1/1 -> Discrete differentiator2/1
  Gain2/1 -> Rate Transition/1

== system vvc1phase_simpower/SensorSigProc_Sinc3_N2048_153p6us2 ==
  note: Sinc3, N=2048, 20MHz to 9.7kHz, settling time = 3*2048*0.05e-6=307.2us, delay=153.6us
  Input : Inport
  Discrete Integrator : DiscreteFilter  Denominator=[1 -1]
  Discrete Integrator1 : DiscreteFilter  Denominator=[1 -1]
  Discrete Integrator2 : DiscreteFilter  Denominator=[1 -1]
  Discrete differentiator : DiscreteFilter  Numerator=[1 -1]  Denominator=[1]
  Discrete differentiator1 : DiscreteFilter  Numerator=[1 -1]  Denominator=[1]
  Discrete differentiator2 : DiscreteFilter  Numerator=[1 -1]  Denominator=[1]
  Gain : Gain  Gain=1/2048
  Gain1 : Gain  Gain=1/2048
  Gain2 : Gain  Gain=1/2048
  Rate Transition : RateTransition
  Zero-Order Hold : ZeroOrderHold  SampleTime=2048*0.05e-6
  Zero-Order Hold2 : ZeroOrderHold  SampleTime=.00000005
  Output : Outport
  wires:
  Gain2/1 -> Rate Transition/1
  Gain1/1 -> Discrete differentiator2/1
  Gain/1 -> Discrete differentiator1/1
  Input/1 -> Discrete Integrator/1
  Discrete Integrator/1 -> Discrete Integrator1/1
  Discrete Integrator1/1 -> Discrete Integrator2/1
  Discrete Integrator2/1 -> Zero-Order Hold/1
  Zero-Order Hold/1 -> Discrete differentiator/1
  Discrete differentiator/1 -> Gain/1
  Discrete differentiator1/1 -> Gain1/1
  Discrete differentiator2/1 -> Gain2/1
  Zero-Order Hold2/1 -> Output/1
  Rate Transition/1 -> Zero-Order Hold2/1

== system vvc1phase_simpower/SensorSigProc_Sinc3_N2048_153p6us3 ==
  note: Sinc3, N=2048, 20MHz to 9.7kHz, settling time = 3*2048*0.05e-6=307.2us, delay=153.6us
  Input : Inport
  Discrete Integrator : DiscreteFilter  Denominator=[1 -1]
  Discrete Integrator1 : DiscreteFilter  Denominator=[1 -1]
  Discrete Integrator2 : DiscreteFilter  Denominator=[1 -1]
  Discrete differentiator : DiscreteFilter  Numerator=[1 -1]  Denominator=[1]
  Discrete differentiator1 : DiscreteFilter  Numerator=[1 -1]  Denominator=[1]
  Discrete differentiator2 : DiscreteFilter  Numerator=[1 -1]  Denominator=[1]
  Gain : Gain  Gain=1/2048
  Gain1 : Gain  Gain=1/2048
  Gain2 : Gain  Gain=1/2048
  Rate Transition : RateTransition
  Zero-Order Hold : ZeroOrderHold  SampleTime=2048*0.05e-6
  Zero-Order Hold2 : ZeroOrderHold  SampleTime=.00000005
  Output : Outport
  wires:
  Gain2/1 -> Rate Transition/1
  Gain1/1 -> Discrete differentiator2/1
  Gain/1 -> Discrete differentiator1/1
  Input/1 -> Discrete Integrator/1
  Discrete Integrator/1 -> Discrete Integrator1/1
  Discrete Integrator1/1 -> Discrete Integrator2/1
  Discrete Integrator2/1 -> Zero-Order Hold/1
  Zero-Order Hold/1 -> Discrete differentiator/1
  Discrete differentiator/1 -> Gain/1
  Discrete differentiator1/1 -> Gain1/1
  Discrete differentiator2/1 -> Gain2/1
  Zero-Order Hold2/1 -> Output/1
  Rate Transition/1 -> Zero-Order Hold2/1
